simulink model "Part1_Simulink"  (R2020a)
settings: Solver=FixedStepAuto  StartTime=0.0  StopTime=inf  FixedStep=1e-3  RelTol=1e-3  EnableMultiTasking=on
undefined symbols (not defined in the file): A0, A1, D0, D1, D10, D11, D12, D13, D2, D3, D4, D5, D6, D7, D8, D9, PTA0, PTA1, PTA2, PTB2, PTB23, PTB3, PTB9, PTC16, PTC17, PTC2, PTC3, PTC4, PTD0, PTD1, PTD2, PTD3
libraries: frdmk64flib x22, nucleoutilitieslib x17
settings Model: ExtModeTrigDuration=5  Creator=kathr  LastModifiedBy=kathr
settings OptimizationCC: EnhancedBackFolding=on  PassReuseOutputArgsAs=Individual arguments  ZeroExternalMemoryAtStartup=off  ZeroInternalMemoryAtStartup=off  MaxStackSize=64  OptimizeBlockOrder=speed  DifferentSizesBufferReuse=on  OptimizationCustomize=off  EfficientTunableParamExpr=on
settings DebuggingCC: ParameterTunabilityLossMsg=error
settings HardwareCC: ProdBitPerPointer=32  ProdBitPerSizeT=32  ProdBitPerPtrDiffT=32  ProdLargestAtomicInteger=Long  ProdLargestAtomicFloat=Double  ProdWordSize=32  ProdHWDeviceType=ARM Compatible->ARM Cortex
settings SFSimCC: MATLABDynamicMemAlloc=off
settings RTWCC: SystemTargetFile=ert.tlc  HardwareBoard=NXP FRDM-K64F  TemplateMakefile=ert_default_tmf  Toolchain=GNU Tools for ARM Embedded Processors
settings CodeAppCC: ForceParamTrailComments=on  IgnoreCustomStorageClasses=off  OperatorAnnotations=on  SimulinkDataObjDesc=on  SFDataObjDesc=on  InsertBlockDesc=on

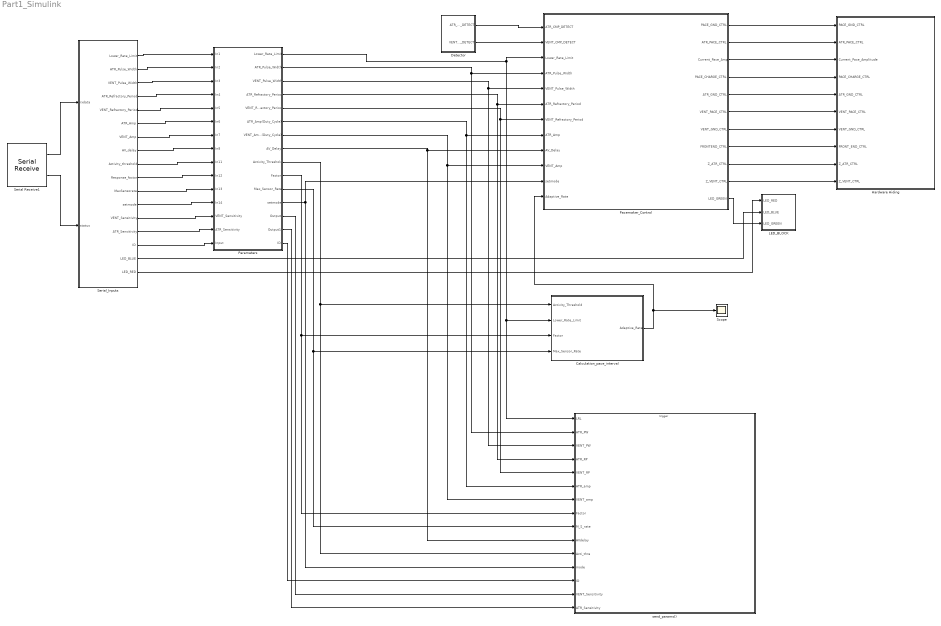
== system Part1_Simulink ==
  Calculation_pace_interval : Subsystem
  Detector : Subsystem
  Hardware Hiding : Subsystem
  LED_BLOCK : Subsystem
  Pacemaker_Control : Stateflow chart  TreatAsAtomicUnit=on
  Parameters : Subsystem
  Scope : Scope
  Serial Receive1 : frdmk64flib/Serial Receive  SCIModule=0  Baudrate=uint32(9600)  Parity=None  StopBits=1  HardwareFlowControl=None  ByteOrder=LittleEndian  DataType=uint8  DataLength=42  BlockingMode=off  OutputStatus=on  SampleTime=-1
  Serial_Inputs : Stateflow chart  TreatAsAtomicUnit=on
  "send_params() " : Subsystem
  wires:
  Serial_Inputs/7(VENT_Amp) -> Parameters/7(In7)
  Serial_Inputs/4(ATR_Refractory_Period) -> Parameters/4(In4)
  Pacemaker_Control/4(PACE_CHARGE_CTRL) -> Hardware Hiding/4(PACE_CHARGE_CTRL)
  Serial_Inputs/2(ATR_Pulse_Width) -> Parameters/2(In2)
  Parameters/4(ATR_Refractory_Period) -> "send_params() "/4(ATR_RP), Pacemaker_Control/6(ATR_Refractory_Period)
  Pacemaker_Control/9(Z_ATR_CTRL) -> Hardware Hiding/9(Z_ATR_CTRL)
  Parameters/5(VENT_Refractory_Period) -> "send_params() "/5(VENT_RP), Pacemaker_Control/7(VENT_Refractory_Period)
  Calculation_pace_interval/1(Adaptive_Rate) -> Pacemaker_Control/12(Adaptive_Rate), Scope/1
  Serial_Inputs/3(VENT_Pulse_Width) -> Parameters/3(In3)
  Pacemaker_Control/7(VENT_GND_CTRL) -> Hardware Hiding/7(VENT_GND_CTRL)
  Serial_Inputs/17(LED_RED) -> LED_BLOCK/1(LED_RED)
  Parameters/3(VENT_Pulse_Width) -> "send_params() "/3(VENT_PW), Pacemaker_Control/5(VENT_Pulse_Width)
  Detector/1(ATR_CMP_DETECT) -> Pacemaker_Control/1(ATR_CMP_DETECT)
  Pacemaker_Control/5(ATR_GND_CTRL) -> Hardware Hiding/5(ATR_GND_CTRL)
  Parameters/10(Factor) -> "send_params() "/8(Factor), Calculation_pace_interval/3(Factor)
  Parameters/8(AV_Delay) -> "send_params() "/10(AVdelay), Pacemaker_Control/9(AV_Delay)
  Pacemaker_Control/10(Z_VENT_CTRL) -> Hardware Hiding/10(Z_VENT_CTRL)
  Serial_Inputs/9(Activity_threshold) -> Parameters/9(In11)
  Parameters/1("Lower_Rate_Limit ") -> Pacemaker_Control/3(Lower_Rate_Limit), "send_params() "/1(LRL), Calculation_pace_interval/2(Lower_Rate_Limit)
  Serial_Inputs/5(VENT_Refractory_Period) -> Parameters/5(In5)
  Parameters/7(VENT_Amp(Duty_Cycle)) -> "send_params() "/7(VENT_amp), Pacemaker_Control/10(VENT_Amp)
  Serial_Inputs/11(MaxSensorate) -> Parameters/11(In13)
  Parameters/9(Activity_Threshold) -> "send_params() "/11(Acti_thre), Calculation_pace_interval/1(Activity_Threshold)
  Serial_Inputs/6(ATR_Amp) -> Parameters/6(In6)
  Pacemaker_Control/1(PACE_GND_CTRL) -> Hardware Hiding/1(PACE_GND_CTRL)
  Serial_Inputs/10(Response_factor) -> Parameters/10(In12)
  Serial_Inputs/12(setmode) -> Parameters/12(In14)
  Pacemaker_Control/3(Current_Pace_Amp) -> Hardware Hiding/3(Current_Pace_Amplitude)
  Parameters/11(Max_Sensor_Rate) -> "send_params() "/9(M_S_rate), Calculation_pace_interval/4(Max_Sensor_Rate)
  Pacemaker_Control/6(VENT_PACE_CTRL) -> Hardware Hiding/6(VENT_PACE_CTRL)
  Parameters/6(ATR_Amp(Duty_Cycle)) -> "send_params() "/6(ATR_amp), Pacemaker_Control/8(ATR_Amp)
  Pacemaker_Control/8(FRONTEND_CTRL) -> Hardware Hiding/8(FRONT_END_CTRL)
  Parameters/12("setmode ") -> "send_params() "/12(mode), Pacemaker_Control/11(setmode)
  Serial Receive1/1 -> Serial_Inputs/1(rxdata)
  Serial_Inputs/1(Lower_Rate_Limit) -> Parameters/1(In1)
  Detector/2(VENT_CMP_DETECT) -> Pacemaker_Control/2(VENT_CMP_DETECT)
  Parameters/2(ATR_Pulse_Width) -> "send_params() "/2(ATR_PW), Pacemaker_Control/4(ATR_Pulse_Width)
  Serial_Inputs/8(AV_delay) -> Parameters/8(In8)
  Pacemaker_Control/2(ATR_PACE_CTRL) -> Hardware Hiding/2(ATR_PACE_CTRL)
  Serial_Inputs/13(VENT_Sensitivity) -> Parameters/13(VENT_Sensitivity)
  Serial_Inputs/14(ATR_Sensitivity) -> Parameters/14(ATR_Sensitivity)
  Serial_Inputs/15(ID) -> Parameters/15(Input)
  Parameters/13(Output) -> "send_params() "/14(VENT_Sensitivity)
  Parameters/14(Output1) -> "send_params() "/15(ATR_Sensitivity)
  Parameters/15(ID) -> "send_params() "/13(ID)
  Serial_Inputs/16(LED_BLUE) -> LED_BLOCK/2(LED_BLUE)
  Pacemaker_Control/11(LED_GREEN) -> LED_BLOCK/3(LED_GREEN)
  Serial Receive1/2 -> Serial_Inputs/2(status)

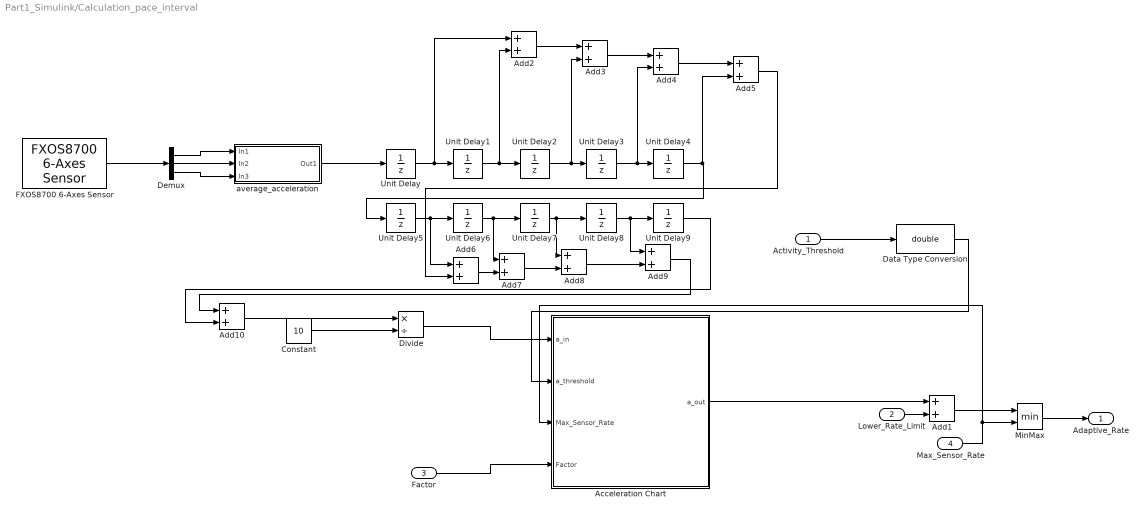
== system Part1_Simulink/Calculation_pace_interval ==
  Activity_Threshold : Inport  OutDataTypeStr=uint16
  Lower_Rate_Limit : Inport  Port=2  OutDataTypeStr=uint16
  Factor : Inport  Port=3  OutDataTypeStr=uint16
  Max_Sensor_Rate : Inport  Port=4  OutDataTypeStr=uint16
  Acceleration Chart : Stateflow chart  TreatAsAtomicUnit=on
  Add{1..10} (10 alike) : Sum
  Constant : Constant  Value=10
  Data Type Conversion : DataTypeConversion  OutDataTypeStr=double
  Demux : Demux  Outputs=3
  Divide : Product  Inputs=*/
  FXOS8700 6-Axes Sensor : frdmk64flib/FXOS8700 6-Axes Sensor  Activesensor=Accelerometer only  ODR=1.5625Hz  HybridODR=400Hz  Accelfullrange=-4g to +4g  SampleTime=0.1
  MinMax : MinMax  Inputs=2
  Unit Delay{,1..9} (10 alike) : UnitDelay  SampleTime=-1  HasFrameUpgradeWarning=on
  average_acceleration : Subsystem
  Adaptive_Rate : Outport  OutDataTypeStr=uint16  VectorParamsAs1DForOutWhenUnconnected=off
  wires:
  Lower_Rate_Limit/1 -> Add1/2
  Acceleration Chart/1(a_out) -> Add1/1
  Activity_Threshold/1 -> Data Type Conversion/1
  Factor/1 -> Acceleration Chart/4(Factor)
  Add1/1 -> MinMax/1
  MinMax/1 -> Adaptive_Rate/1
  Demux/3 -> average_acceleration/3(In3)
  Demux/1 -> average_acceleration/1(In1)
  Demux/2 -> average_acceleration/2(In2)
  FXOS8700 6-Axes Sensor/1 -> Demux/1
  Max_Sensor_Rate/1 -> MinMax/2, Acceleration Chart/3(Max_Sensor_Rate)
  Data Type Conversion/1 -> Acceleration Chart/2(a_threshold)
  Unit Delay1/1 -> Add2/2, Unit Delay2/1
  Unit Delay2/1 -> Add3/2, Unit Delay3/1
  Unit Delay3/1 -> Add4/2, Unit Delay4/1
  Unit Delay4/1 -> Add5/2, Unit Delay5/1
  Unit Delay5/1 -> Add6/1, Unit Delay6/1
  Unit Delay6/1 -> Add7/1, Unit Delay7/1
  Unit Delay7/1 -> Add8/1, Unit Delay8/1
  Unit Delay8/1 -> Add9/1, Unit Delay9/1
  Constant/1 -> Divide/2
  Divide/1 -> Acceleration Chart/1(a_in)
  average_acceleration/1(Out1) -> Unit Delay/1
  Unit Delay/1 -> Add2/1, Unit Delay1/1
  Add2/1 -> Add3/1
  Add3/1 -> Add4/1
  Add4/1 -> Add5/1
  Add5/1 -> Add6/2
  Add6/1 -> Add7/2
  Add8/1 -> Add9/2
  Add10/1 -> Divide/1
  Add9/1 -> Add10/1
  Unit Delay9/1 -> Add10/2
  Add7/1 -> Add8/2

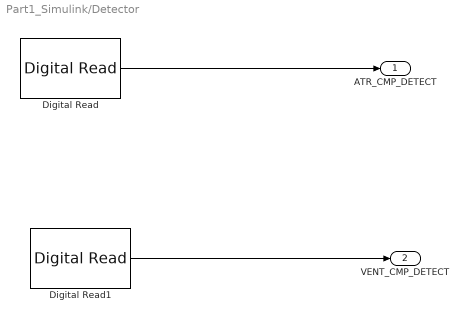
== system Part1_Simulink/Detector ==
  Digital Read : frdmk64flib/Digital Read  Whichpin=PTC16 (D0)  SampleTime=-1
  Digital Read1 : frdmk64flib/Digital Read  Whichpin=PTC17 (D1)  SampleTime=-1
  ATR_CMP_DETECT : Outport  OutDataTypeStr=boolean
  VENT_CMP_DETECT : Outport  Port=2  OutDataTypeStr=boolean
  wires:
  Digital Read/1 -> ATR_CMP_DETECT/1
  Digital Read1/1 -> VENT_CMP_DETECT/1

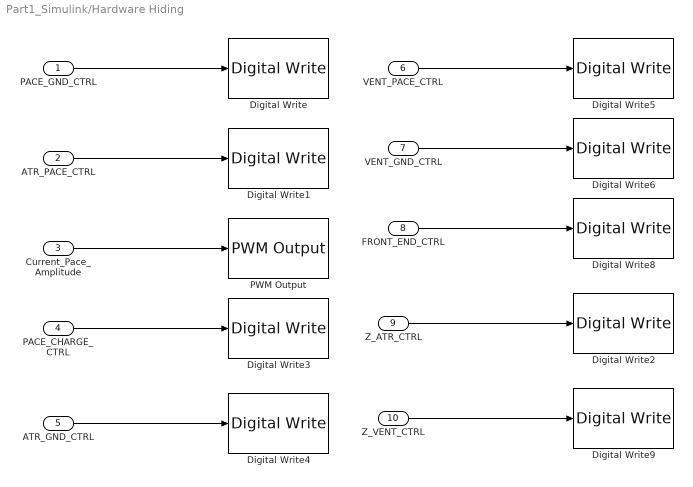
== system Part1_Simulink/Hardware Hiding ==
  PACE_GND_CTRL : Inport  OutDataTypeStr=boolean
  ATR_PACE_CTRL : Inport  Port=2  OutDataTypeStr=boolean
  Current_Pace_Amplitude : Inport  Port=3  OutDataTypeStr=uint16
  PACE_CHARGE_CTRL : Inport  Port=4  OutDataTypeStr=boolean
  ATR_GND_CTRL : Inport  Port=5  OutDataTypeStr=boolean
  VENT_PACE_CTRL : Inport  Port=6  OutDataTypeStr=boolean
  VENT_GND_CTRL : Inport  Port=7  OutDataTypeStr=boolean
  FRONT_END_CTRL : Inport  Port=8  OutDataTypeStr=boolean
  Z_ATR_CTRL : Inport  Port=9  OutDataTypeStr=boolean
  Z_VENT_CTRL : Inport  Port=10  OutDataTypeStr=boolean
  Digital Write : frdmk64flib/Digital Write  Whichpin=PTD0 (D10)
  Digital Write1 : frdmk64flib/Digital Write  Whichpin=PTA0 (D8)
  Digital Write2 : frdmk64flib/Digital Write  Whichpin=PTB23 (D4)
  Digital Write3 : frdmk64flib/Digital Write  Whichpin=PTB9 (D2)
  Digital Write4 : frdmk64flib/Digital Write  Whichpin=PTD2 (D11)
  Digital Write5 : frdmk64flib/Digital Write  Whichpin=PTC4 (D9)
  Digital Write6 : frdmk64flib/Digital Write  Whichpin=PTD3 (D12)
  Digital Write8 : frdmk64flib/Digital Write  Whichpin=PTD1 (D13)
  Digital Write9 : frdmk64flib/Digital Write  Whichpin=PTC3 (D7)
  PWM Output : frdmk64flib/PWM Output  Whichpin=PTA2 (D5)  InitialFrequency=2000  InitialDutyCycle=100
  wires:
  PACE_GND_CTRL/1 -> Digital Write/1
  ATR_PACE_CTRL/1 -> Digital Write1/1
  Current_Pace_Amplitude/1 -> PWM Output/1
  PACE_CHARGE_CTRL/1 -> Digital Write3/1
  ATR_GND_CTRL/1 -> Digital Write4/1
  VENT_PACE_CTRL/1 -> Digital Write5/1
  VENT_GND_CTRL/1 -> Digital Write6/1
  FRONT_END_CTRL/1 -> Digital Write8/1
  Z_VENT_CTRL/1 -> Digital Write9/1
  Z_ATR_CTRL/1 -> Digital Write2/1

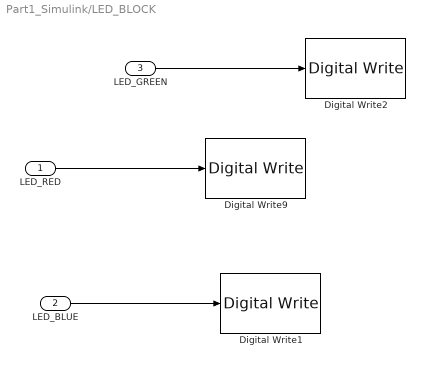
== system Part1_Simulink/LED_BLOCK ==
  LED_RED : Inport  OutDataTypeStr=boolean
  LED_BLUE : Inport  Port=2  OutDataTypeStr=boolean
  LED_GREEN : Inport  Port=3  OutDataTypeStr=boolean
  Digital Write1 : frdmk64flib/Digital Write  Whichpin=BLUE_LED
  Digital Write2 : frdmk64flib/Digital Write  Whichpin=GREEN_LED
  Digital Write9 : frdmk64flib/Digital Write  Whichpin=RED_LED
  wires:
  LED_RED/1 -> Digital Write9/1
  LED_BLUE/1 -> Digital Write1/1
  LED_GREEN/1 -> Digital Write2/1

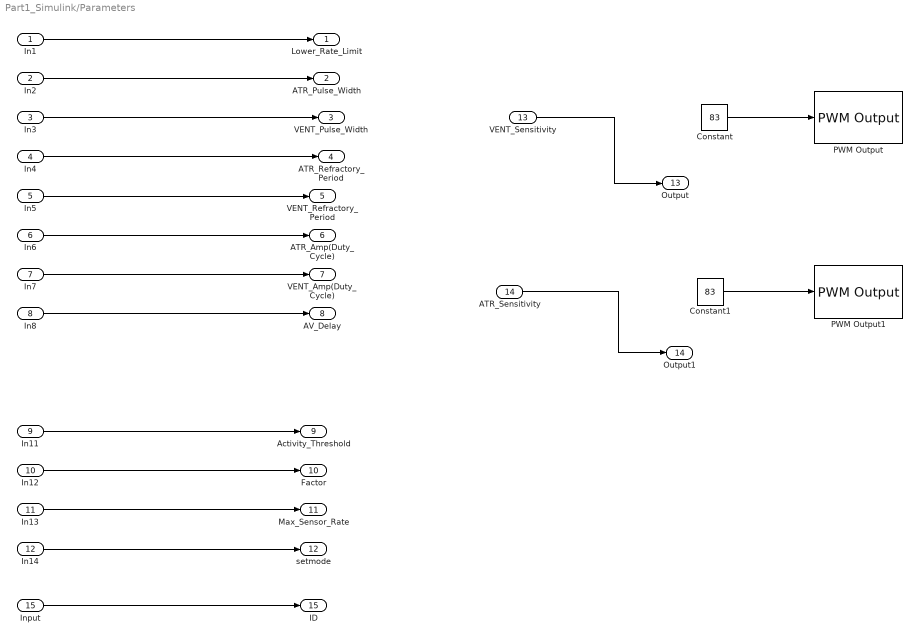
== system Part1_Simulink/Parameters ==
  In1 : Inport
  In2 : Inport  Port=2
  In3 : Inport  Port=3
  In4 : Inport  Port=4
  In5 : Inport  Port=5
  In6 : Inport  Port=6
  In7 : Inport  Port=7
  In8 : Inport  Port=8
  In11 : Inport  Port=9
  In12 : Inport  Port=10
  In13 : Inport  Port=11
  In14 : Inport  Port=12
  VENT_Sensitivity : Inport  Port=13
  ATR_Sensitivity : Inport  Port=14
  Input : Inport  Port=15
  Constant : Constant  Value=83
  Constant1 : Constant  Value=83
  PWM Output : frdmk64flib/PWM Output  Whichpin=PTC2 (D6)  InitialFrequency=2000  InitialDutyCycle=75
  PWM Output1 : frdmk64flib/PWM Output  Whichpin=PTA1 (D3)  InitialFrequency=2000  InitialDutyCycle=100
  "Lower_Rate_Limit " : Outport  OutDataTypeStr=uint16
  ATR_Pulse_Width : Outport  Port=2  OutDataTypeStr=uint16
  VENT_Pulse_Width : Outport  Port=3  OutDataTypeStr=uint16
  ATR_Refractory_Period : Outport  Port=4  OutDataTypeStr=uint16
  VENT_Refractory_Period : Outport  Port=5  OutDataTypeStr=uint16
  ATR_Amp(Duty_Cycle) : Outport  Port=6  OutDataTypeStr=uint16
  VENT_Amp(Duty_Cycle) : Outport  Port=7  OutDataTypeStr=uint16
  AV_Delay : Outport  Port=8  OutDataTypeStr=uint16
  Activity_Threshold : Outport  Port=9  OutDataTypeStr=uint16
  Factor : Outport  Port=10  OutDataTypeStr=uint16
  Max_Sensor_Rate : Outport  Port=11  OutDataTypeStr=uint16
  "setmode " : Outport  Port=12  VectorParamsAs1DForOutWhenUnconnected=off
  Output : Outport  Port=13
  Output1 : Outport  Port=14
  ID : Outport  Port=15
  wires:
  In5/1 -> VENT_Refractory_Period/1
  In2/1 -> ATR_Pulse_Width/1
  In4/1 -> ATR_Refractory_Period/1
  In6/1 -> ATR_Amp(Duty_Cycle)/1
  In7/1 -> VENT_Amp(Duty_Cycle)/1
  In3/1 -> VENT_Pulse_Width/1
  In1/1 -> "Lower_Rate_Limit "/1
  In8/1 -> AV_Delay/1
  In11/1 -> Activity_Threshold/1
  In12/1 -> Factor/1
  In13/1 -> Max_Sensor_Rate/1
  In14/1 -> "setmode "/1
  Input/1 -> ID/1
  VENT_Sensitivity/1 -> Output/1
  ATR_Sensitivity/1 -> Output1/1
  Constant/1 -> PWM Output/1
  Constant1/1 -> PWM Output1/1

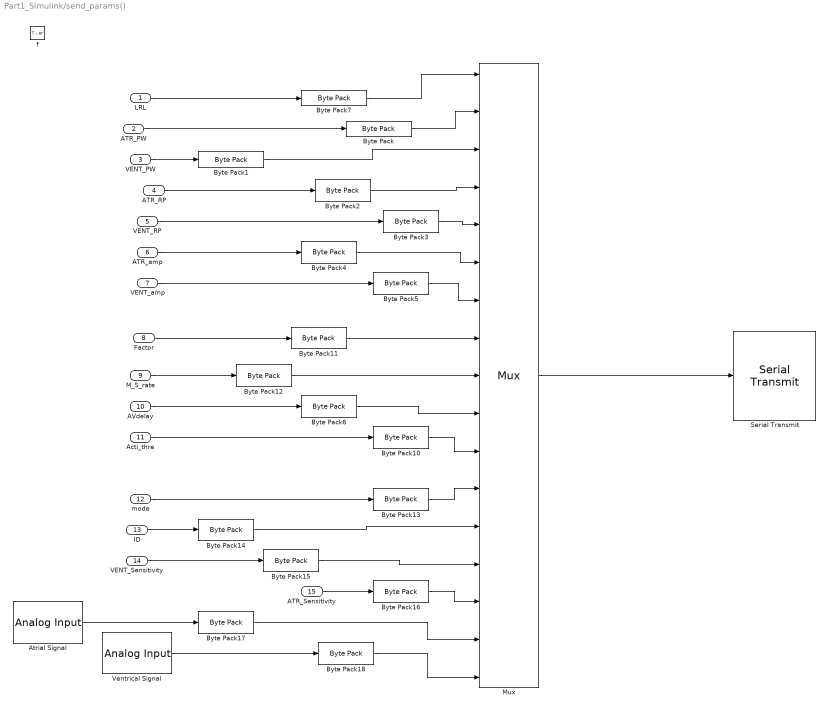
== system Part1_Simulink/send_params()  ==
  LRL : Inport  OutDataTypeStr=uint16
  ATR_PW : Inport  Port=2  OutDataTypeStr=uint16
  VENT_PW : Inport  Port=3  OutDataTypeStr=uint16
  ATR_RP : Inport  Port=4  OutDataTypeStr=uint16
  VENT_RP : Inport  Port=5  OutDataTypeStr=uint16
  ATR_amp : Inport  Port=6  OutDataTypeStr=uint16
  VENT_amp : Inport  Port=7  OutDataTypeStr=uint16
  Factor : Inport  Port=8  OutDataTypeStr=uint16
  M_S_rate : Inport  Port=9  OutDataTypeStr=uint16
  AVdelay : Inport  Port=10  OutDataTypeStr=uint16
  Acti_thre : Inport  Port=11  OutDataTypeStr=uint16
  mode : Inport  Port=12  OutDataTypeStr=uint16
  ID : Inport  Port=13  OutDataTypeStr=uint16
  VENT_Sensitivity : Inport  Port=14  OutDataTypeStr=double
  ATR_Sensitivity : Inport  Port=15  OutDataTypeStr=double
  f : TriggerPort  TriggerType=function-call  IsSimulinkFunction=on  FunctionName=send_params  VariantControl=(inherit)
  Atrial Signal : frdmk64flib/Analog Input  Whichpin=PTB2 (A0)  SampleTime=-1
  Byte Pack{,1..7,10..14} (13 alike) : nucleoutilitieslib/Byte Pack  datatypes={'uint16'}  byteAlign=1  blockPlatform=nucleo
      settings: SourceProductBaseCode=ARDUINO,ML_ARDUINO,ECCORTEXA,ECCORTEXR,SC_BEAGLEBONE_BLUE,EC_FREEDOM_BOARD,EC_FRDM_K64F,INTEL_BLOCKSET,MICROBIT,NUCLEO,PX4AUTOPILOTS,RASPPIIO,STMICRODIS,TIC2000,XILINX_BLOCKSET
  Byte Pack{15..18} (4 alike) : nucleoutilitieslib/Byte Pack  datatypes={'double'}  byteAlign=1  blockPlatform=nucleo
      settings: SourceProductBaseCode=ARDUINO,ML_ARDUINO,ECCORTEXA,ECCORTEXR,SC_BEAGLEBONE_BLUE,EC_FREEDOM_BOARD,EC_FRDM_K64F,INTEL_BLOCKSET,MICROBIT,NUCLEO,PX4AUTOPILOTS,RASPPIIO,STMICRODIS,TIC2000,XILINX_BLOCKSET
  Mux : Mux  Inputs=17
  Serial Transmit : frdmk64flib/Serial Transmit  SCIModule=0  Baudrate=uint32(9600)  Parity=None  StopBits=1  HardwareFlowControl=None  ByteOrder=LittleEndian  BlockingMode=on  OutputStatus=off
  Ventrical Signal : frdmk64flib/Analog Input  Whichpin=PTB3 (A1)  SampleTime=-1
  wires:
  LRL/1 -> Byte Pack7/1
  VENT_PW/1 -> Byte Pack1/1
  ATR_RP/1 -> Byte Pack2/1
  Mux/1 -> Serial Transmit/1
  ATR_amp/1 -> Byte Pack4/1
  VENT_RP/1 -> Byte Pack3/1
  VENT_amp/1 -> Byte Pack5/1
  ATR_PW/1 -> Byte Pack/1
  Byte Pack/1 -> Mux/2
  Byte Pack1/1 -> Mux/3
  Byte Pack2/1 -> Mux/4
  Byte Pack3/1 -> Mux/5
  Byte Pack4/1 -> Mux/6
  Byte Pack5/1 -> Mux/7
  Byte Pack7/1 -> Mux/1
  AVdelay/1 -> Byte Pack6/1
  Acti_thre/1 -> Byte Pack10/1
  Factor/1 -> Byte Pack11/1
  M_S_rate/1 -> Byte Pack12/1
  mode/1 -> Byte Pack13/1
  ID/1 -> Byte Pack14/1
  VENT_Sensitivity/1 -> Byte Pack15/1
  ATR_Sensitivity/1 -> Byte Pack16/1
  Atrial Signal/1 -> Byte Pack17/1
  Ventrical Signal/1 -> Byte Pack18/1
  Byte Pack11/1 -> Mux/8
  Byte Pack12/1 -> Mux/9
  Byte Pack6/1 -> Mux/10
  Byte Pack10/1 -> Mux/11
  Byte Pack13/1 -> Mux/12
  Byte Pack14/1 -> Mux/13
  Byte Pack15/1 -> Mux/14
  Byte Pack16/1 -> Mux/15
  Byte Pack17/1 -> Mux/16
  Byte Pack18/1 -> Mux/17

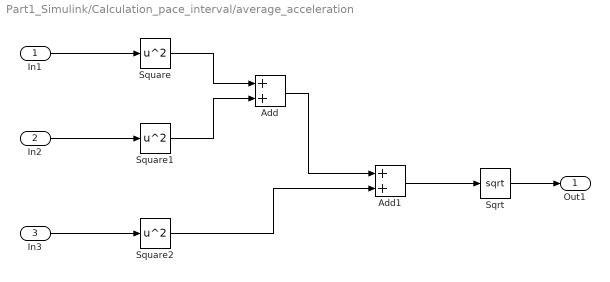
== system Part1_Simulink/Calculation_pace_interval/average_acceleration ==
  In1 : Inport
  In2 : Inport  Port=2
  In3 : Inport  Port=3
  Add : Sum
  Add1 : Sum
  Sqrt : Sqrt  SaturateOnIntegerOverflow=on
  Square : Math  Operator=square  SignedPower=on  SaturateOnIntegerOverflow=on
  Square1 : Math  Operator=square  SignedPower=on  SaturateOnIntegerOverflow=on
  Square2 : Math  Operator=square  SignedPower=on  SaturateOnIntegerOverflow=on
  Out1 : Outport
  wires:
  In1/1 -> Square/1
  In2/1 -> Square1/1
  In3/1 -> Square2/1
  Square/1 -> Add/1
  Square1/1 -> Add/2
  Add/1 -> Add1/1
  Square2/1 -> Add1/2
  Add1/1 -> Sqrt/1
  Sqrt/1 -> Out1/1

== stateflow chart Part1_Simulink/Calculation_pace_interval/Acceleration Chart ==
  state LOW_TO_MID
    entry:
    if(a_out+Factor<=Max_Sensor_Rate/2)
    a_out = a_out + Factor;
    end
  state MID
    entry:
    %LED_BLUE = true;
  state LOW
    entry:
    a_out = 0;
    %LED_RED = true;
  state MID_TO_HIGH
    entry:
    if(a_out+Factor <=Max_Sensor_Rate)
    a_out = a_out+Factor;
    end
  state LOW_TO_HIGH
    entry:
    if(a_out+Factor+Factor <=Max_Sensor_Rate)
    a_out = a_out+Factor+Factor;
    end
  state HIGH_TO_MID
    entry:
    a_out = a_out-Factor;
  state HIGH
    entry:
    %LED_BLUE = true;
  LOW_TO_MID -> MID
  LOW -> LOW_TO_MID [order 2] : [a_in<=(1+a_threshold/10) && a_in>(1+a_threshold/20)]
  MID -> MID [order 1] : [a_in<=(1+a_threshold/10) && a_in>(1+a_threshold/20)]
  HIGH_TO_MID -> MID
  (default) -> LOW
  MID -> LOW [order 2] : [a_in<=(1+a_threshold/20)]
  MID -> MID_TO_HIGH [order 3] : [a_in>(1+a_threshold/10)]
  LOW -> LOW [order 1] : [a_in<=(1+a_threshold/20)]
  LOW -> LOW_TO_HIGH [order 3] : [a_in>(1+a_threshold/10)]
  HIGH -> LOW [order 2] : [a_in<=(1+a_threshold/20)]
  MID_TO_HIGH -> HIGH
  HIGH -> HIGH [order 1] : [a_in>(1+a_threshold/10)]
  LOW_TO_HIGH -> HIGH
  HIGH -> HIGH_TO_MID [order 3] : [a_in<=(1+a_threshold/5) && a_in>(1+a_threshold/20)]
  data: a_in input double; a_out output uint16; a_threshold input double; Max_Sensor_Rate input uint16; Factor input uint16

== stateflow chart Part1_Simulink/Pacemaker_Control ==
  state AOO
    entry:
    PACE_CHARGE_CTRL=false;
    VENT_PACE_CTRL=false;
    PACE_CHARGE_CTRL=true;
    PACE_GND_CTRL=true;
    VENT_PACE_CTRL=false;
    Z_ATR_CTRL=false;
    Z_VENT_CTRL=false;
    ATR_PACE_CTRL=false;
    ATR_GND_CTRL=true;
    VENT_GND_CTRL=false;
    %LED_GREEN=false;
  state AOO_PACE
    entry:
    PACE_CHARGE_CTRL=false;
    PACE_GND_CTRL=true;
    ATR_PACE_CTRL=true;
    ATR_GND_CTRL=false;
    Z_ATR_CTRL=false;
    Z_VENT_CTRL=false;
    VENT_GND_CTRL=false;
    VENT_PACE_CTRL=false;
    %LED_GREEN=true;
    Current_Pace_Amp=ATR_Amp;
  state AOOR
    entry:
    PACE_CHARGE_CTRL=false;
    VENT_PACE_CTRL=false;
    PACE_CHARGE_CTRL=true;
    PACE_GND_CTRL=true;
    VENT_PACE_CTRL=false;
    Z_ATR_CTRL=false;
    Z_VENT_CTRL=false;
    ATR_PACE_CTRL=false;
    ATR_GND_CTRL=true;
    VENT_GND_CTRL=false;
    LED_GREEN=false;
  state pacing_AOOR
    entry:
    PACE_CHARGE_CTRL=false;
    PACE_GND_CTRL=true;
    ATR_PACE_CTRL=true;
    ATR_GND_CTRL=false;
    Z_ATR_CTRL=false;
    Z_VENT_CTRL=false;
    VENT_GND_CTRL=false;
    VENT_PACE_CTRL=false;
    LED_GREEN=true;
    Current_Pace_Amp=ATR_Amp;
  state VOO_PACE
    entry:
    PACE_CHARGE_CTRL=false;
    PACE_GND_CTRL=true;
    ATR_PACE_CTRL=false;
    ATR_GND_CTRL=false;
    Z_ATR_CTRL=false;
    Z_VENT_CTRL=false;
    VENT_GND_CTRL=false;
    VENT_PACE_CTRL=true;
    %LED_GREEN=true;
    Current_Pace_Amp = VENT_Amp;
  state VOO
    entry:
    PACE_CHARGE_CTRL=false;
    VENT_PACE_CTRL=false;
    PACE_CHARGE_CTRL=true;
    PACE_GND_CTRL=true;
    VENT_PACE_CTRL=false;
    Z_ATR_CTRL=false;
    Z_VENT_CTRL=false;
    ATR_PACE_CTRL=false;
    ATR_GND_CTRL=false;
    VENT_GND_CTRL=true;
    %LED_GREEN=false;
  state VOOR
    entry:
    PACE_CHARGE_CTRL=false;
    VENT_PACE_CTRL=false;
    PACE_CHARGE_CTRL=true;
    PACE_GND_CTRL=true;
    VENT_PACE_CTRL=false;
    Z_ATR_CTRL=false;
    Z_VENT_CTRL=false;
    ATR_PACE_CTRL=false;
    ATR_GND_CTRL=false;
    VENT_GND_CTRL=true;
    LED_GREEN=false;
  state pacing_VOOR
    entry:
    PACE_CHARGE_CTRL=false;
    PACE_GND_CTRL=true;
    ATR_PACE_CTRL=false;
    ATR_GND_CTRL=false;
    Z_ATR_CTRL=false;
    Z_VENT_CTRL=false;
    VENT_GND_CTRL=false;
    VENT_PACE_CTRL=true;
    LED_GREEN=true;
    Current_Pace_Amp = VENT_Amp;
  state AAI_PACE
    entry:
    FRONTEND_CTRL=false;
    PACE_CHARGE_CTRL=false;
    PACE_GND_CTRL=true;
    ATR_PACE_CTRL=true;
    ATR_GND_CTRL=false;
    Z_ATR_CTRL=false;
    Z_VENT_CTRL=false;
    VENT_GND_CTRL=false;
    VENT_PACE_CTRL=false;
    %LED_GREEN=true;
    Current_Pace_Amp=ATR_Amp;
  state AAI
    entry:
    FRONTEND_CTRL=false;
    PACE_CHARGE_CTRL=false;
    VENT_PACE_CTRL=false;
    PACE_CHARGE_CTRL=true;
    PACE_GND_CTRL=true;
    VENT_PACE_CTRL=false;
    Z_ATR_CTRL=false;
    Z_VENT_CTRL=false;
    ATR_PACE_CTRL=false;
    ATR_GND_CTRL=true;
    VENT_GND_CTRL=false;
    %LED_GREEN=false;
  state AAI_REF_PERIOD1
    entry:
    FRONTEND_CTRL=true;
    PACE_CHARGE_CTRL=true;
    PACE_GND_CTRL=true;
    ATR_PACE_CTRL=false;
    ATR_GND_CTRL=true;
    Z_ATR_CTRL=false;
    Z_VENT_CTRL=false;
    VENT_GND_CTRL=false;
    VENT_PACE_CTRL=false;
    %LED_GREEN=true;
    Current_Pace_Amp=ATR_Amp;
  state pacing_AAIR
    entry:
    FRONTEND_CTRL=false;
    PACE_CHARGE_CTRL=false;
    PACE_GND_CTRL=true;
    ATR_PACE_CTRL=true;
    ATR_GND_CTRL=false;
    Z_ATR_CTRL=false;
    Z_VENT_CTRL=false;
    VENT_GND_CTRL=false;
    VENT_PACE_CTRL=false;
    %LED_GREEN=true;
    Current_Pace_Amp=ATR_Amp;
  state AAIR
    entry:
    FRONTEND_CTRL=false;
    PACE_CHARGE_CTRL=false;
    VENT_PACE_CTRL=false;
    PACE_CHARGE_CTRL=true;
    PACE_GND_CTRL=true;
    VENT_PACE_CTRL=false;
    Z_ATR_CTRL=false;
    Z_VENT_CTRL=false;
    ATR_PACE_CTRL=false;
    ATR_GND_CTRL=true;
    VENT_GND_CTRL=false;
    %LED_GREEN=false;
  state AAI_REF_LED1
    entry:
    %LED_GREEN=false;
  state AAIR_LED1
    entry:
    %LED_GREEN=false;
  state AAI_REF_PERIOD
    entry:
    FRONTEND_CTRL=true;
    PACE_CHARGE_CTRL=true;
    PACE_GND_CTRL=true;
    ATR_PACE_CTRL=false;
    ATR_GND_CTRL=true;
    Z_ATR_CTRL=false;
    Z_VENT_CTRL=false;
    VENT_GND_CTRL=false;
    VENT_PACE_CTRL=false;
    %LED_GREEN=true;
    Current_Pace_Amp=ATR_Amp;
  state Refractory_AAIR1
    entry:
    FRONTEND_CTRL=true;
    PACE_CHARGE_CTRL=true;
    PACE_GND_CTRL=true;
    ATR_PACE_CTRL=false;
    ATR_GND_CTRL=true;
    Z_ATR_CTRL=false;
    Z_VENT_CTRL=false;
    VENT_GND_CTRL=false;
    VENT_PACE_CTRL=false;
    %LED_GREEN=true;
    Current_Pace_Amp=ATR_Amp
  state AAI_REF_LED
    entry:
    %LED_GREEN=false;
  state MAIN
    entry:
    %stop sensing
    FRONTEND_CTRL=false;
    Current_Pace_Amp=0;
  state VVI
    entry:
    FRONTEND_CTRL=false;
    PACE_CHARGE_CTRL=false;
    VENT_PACE_CTRL=false;
    PACE_CHARGE_CTRL=true;
    PACE_GND_CTRL=true;
    VENT_PACE_CTRL=false;
    Z_ATR_CTRL=false;
    Z_VENT_CTRL=false;
    ATR_PACE_CTRL=false;
    ATR_GND_CTRL=false;
    VENT_GND_CTRL=true;
    LED_GREEN=false;
  state Refractory_AAIR
    entry:
    FRONTEND_CTRL=true;
    PACE_CHARGE_CTRL=true;
    PACE_GND_CTRL=true;
    ATR_PACE_CTRL=false;
    ATR_GND_CTRL=true;
    Z_ATR_CTRL=false;
    Z_VENT_CTRL=false;
    VENT_GND_CTRL=false;
    VENT_PACE_CTRL=false;
    %LED_GREEN=true;
    Current_Pace_Amp=ATR_Amp
  state VVI_PACE
    entry:
    FRONTEND_CTRL=false;
    PACE_CHARGE_CTRL=false;
    PACE_GND_CTRL=true;
    ATR_PACE_CTRL=false;
    ATR_GND_CTRL=false;
    Z_ATR_CTRL=false;
    Z_VENT_CTRL=false;
    VENT_GND_CTRL=false;
    VENT_PACE_CTRL=true;
    LED_GREEN=true;
    Current_Pace_Amp = VENT_Amp;
  note: MODE
      | NUMBER
      |
      | VOO
      | 0
      |
      | AOO
      | 1
      |
      | VVI
      | 2
      |
      | AAI
      | 3
      |
      | DOO
      | 4
      |
      | VOOR
      | 5
      |
      | AOOR
      | 6
      |
      | VVIR
      | 7
      |
      | AAIR
      | 8
      |
      | DOOR
      | 9
  state AAIR_LED
    entry:
    %LED_GREEN=false;
  state VVIR
    entry:
    FRONTEND_CTRL=false;
    PACE_CHARGE_CTRL=false;
    VENT_PACE_CTRL=false;
    PACE_CHARGE_CTRL=true;
    PACE_GND_CTRL=true;
    VENT_PACE_CTRL=false;
    Z_ATR_CTRL=false;
    Z_VENT_CTRL=false;
    ATR_PACE_CTRL=false;
    ATR_GND_CTRL=false;
    VENT_GND_CTRL=true;
    %LED_GREEN=false;
  state pacing_VVIR
    entry:
    FRONTEND_CTRL=false;
    PACE_CHARGE_CTRL=false;
    PACE_GND_CTRL=true;
    ATR_PACE_CTRL=false;
    ATR_GND_CTRL=false;
    Z_ATR_CTRL=false;
    Z_VENT_CTRL=false;
    VENT_GND_CTRL=false;
    VENT_PACE_CTRL=true;
    %LED_GREEN=true;
    Current_Pace_Amp = VENT_Amp;
  state VVI_REF_PERIOD2
    entry:
    FRONTEND_CTRL=true;
    PACE_CHARGE_CTRL=true;
    PACE_GND_CTRL=true;
    ATR_PACE_CTRL=false;
    ATR_GND_CTRL=false;
    Z_ATR_CTRL=false;
    Z_VENT_CTRL=false;
    VENT_GND_CTRL=true;
    VENT_PACE_CTRL=false;
    Current_Pace_Amp = VENT_Amp;
    LED_GREEN=false;
  state VVIR_REF_PERIOD2
    %LED_GREEN=false;
  state VVI_LED1
    entry:
    LED_GREEN=true;
  state VVI_REF_PERIOD1
    entry:
    FRONTEND_CTRL=true;
    PACE_CHARGE_CTRL=true;
    PACE_GND_CTRL=true;
    ATR_PACE_CTRL=false;
    ATR_GND_CTRL=false;
    Z_ATR_CTRL=false;
    Z_VENT_CTRL=false;
    VENT_GND_CTRL=true;
    VENT_PACE_CTRL=false;
    Current_Pace_Amp = VENT_Amp;
    LED_GREEN=false;
  state Refractory_VVIR1
    entry:
    FRONTEND_CTRL=true;
    PACE_CHARGE_CTRL=true;
    PACE_GND_CTRL=true;
    ATR_PACE_CTRL=false;
    ATR_GND_CTRL=false;
    Z_ATR_CTRL=false;
    Z_VENT_CTRL=false;
    VENT_GND_CTRL=true;
    VENT_PACE_CTRL=false;
    %LED_GREEN=true;
    Current_Pace_Amp = VENT_Amp;
  state Refractory_VVIR
    entry:
    FRONTEND_CTRL=true;
    PACE_CHARGE_CTRL=true;
    PACE_GND_CTRL=true;
    ATR_PACE_CTRL=false;
    ATR_GND_CTRL=false;
    Z_ATR_CTRL=false;
    Z_VENT_CTRL=false;
    VENT_GND_CTRL=true;
    VENT_PACE_CTRL=false;
    %LED_GREEN=true;
    Current_Pace_Amp = VENT_Amp;
  state VVI_LED
    entry:
    LED_GREEN=true;
  note: Discharge C22 to C21 to pace ATR
  state pacing_DOO_ATR
    entry:
    %discharge C22 and charge C21
    PACE_CHARGE_CTRL=false;%disconnect 4
    %connect C22 and C21
    ATR_GND_CTRL = false;
    VENT_GND_CTRL=false;%disconnect 7
    VENT_PACE_CTRL=false;
    ATR_PACE_CTRL=true;%connect 6 for ATR
    PACE_GND_CTRL=true;
    Current_Pace_Amp = ATR_Amp;
    %LED_RED=false;
  state VVIR_REF_PERIOD1
    %LED_GREEN=false;
  note: Charge C22, discharge C21 for VENT
  state DOO
    entry:
    FRONTEND_CTRL=false;
    VENT_PACE_CTRL=false %turn off VENT
    ATR_PACE_CTRL=false;%disconnect 6
    %discharge C21 for VENT
    VENT_GND_CTRL=true;
    PACE_GND_CTRL=true;%connect 10
    ATR_GND_CTRL=false;
    %charge C22
    PACE_CHARGE_CTRL=true;%connect 4
    %set the atrium pacing amplitude
    Current_Pace_Amp = ATR_Amp;
    %LED_RED=true;%use red LED for debugging
    %LED_GREEN=false;
  state pacing_DOOR_ATR
    entry:
    %discharge C22 and charge C21
    PACE_CHARGE_CTRL=false;%disconnect 4
    %connect C22 and C21
    ATR_GND_CTRL = false;
    VENT_GND_CTRL=false;%disconnect 7
    VENT_PACE_CTRL=false;
    ATR_PACE_CTRL=true;%connect 6 for ATR
    PACE_GND_CTRL=true;
    Current_Pace_Amp = ATR_Amp;
    %LED_RED=false;
  state DOOR
    entry:
    FRONTEND_CTRL=false;
    VENT_PACE_CTRL=false; %turn off VENT
    ATR_PACE_CTRL=false;%disconnect 6
    %discharge C21 for VENT
    VENT_GND_CTRL=true;
    PACE_GND_CTRL=true;%connect 10
    ATR_GND_CTRL=false;
    %charge C22
    PACE_CHARGE_CTRL=true;%connect 4
    %set the atrium pacing amplitude
    Current_Pace_Amp = ATR_Amp;
    %LED_RED=true;%use red LED for debugging
  state DOO_VENT
    entry:
    PACE_CHARGE_CTRL=false;%disconnect 4
    PACE_GND_CTRL=true;%connect 10
    VENT_GND_CTRL=false;
    VENT_PACE_CTRL=true;%connect 6
    ATR_GND_CTRL=false;%disconnect 7
    %set the ventricle pacing amplitude
    Current_Pace_Amp = VENT_Amp;
    %LED_GREEN=false;%use red LED for debugging
  state DOO_Vcharge_Adischarge
    entry:
    PACE_CHARGE_CTRL=true;%connect 4
    %disconnect C21 with C22
    ATR_PACE_CTRL=false;%disconnect 6
    VENT_PACE_CTRL=false;
    %discharge C21
    ATR_GND_CTRL=true;%connect 7
    PACE_GND_CTRL=true;%connect 10
    VENT_GND_CTRL=false;
    %set the atrium pacing amplitude
    Current_Pace_Amp = VENT_Amp;
    %LED_GREEN=false;%use green LED for debugging
  note: Discharge C22 to C21 to pace VENT
  note: Charge C22, discharge C21 for ATR
  state DOOR_Vcharge_Adischarge
    entry:
    PACE_CHARGE_CTRL=true;%connect 4
    %disconnect C21 with C22
    ATR_PACE_CTRL=false;%disconnect 6
    VENT_PACE_CTRL=false;
    %discharge C21
    ATR_GND_CTRL=true;%connect 7
    PACE_GND_CTRL=true;%connect 10
    VENT_GND_CTRL=false;
    %set the atrium pacing amplitude
    Current_Pace_Amp = VENT_Amp;
    %LED_GREEN=true;%use green LED for debugging
  state DOOR_VENT
    entry:
    PACE_CHARGE_CTRL=false;%disconnect 4
    PACE_GND_CTRL=true;%connect 10
    VENT_GND_CTRL=false;
    VENT_PACE_CTRL=true;%connect 6
    ATR_GND_CTRL=false;%disconnect 7
    %set the ventricle pacing amplitude
    Current_Pace_Amp = VENT_Amp;
    %LED_GREEN=false;%use red LED for debugging
  AOO_PACE -> AOO : after(ATR_Pulse_Width,msec)
  AOO -> MAIN [order 2] : [setmode~=1]
  AOOR -> pacing_AOOR [order 1] : after(60000/Adaptive_Rate - ATR_Pulse_Width,msec)
  AOO -> AOO_PACE [order 1] : after(60000/Lower_Rate_Limit - ATR_Pulse_Width,msec)
  MAIN -> AOO [order 2] : [setmode==1]
  pacing_AOOR -> AOOR : after(ATR_Pulse_Width,msec)
  AOOR -> MAIN [order 2] : [setmode~=6]
  MAIN -> AOOR [order 9] : [setmode==6]
  VOO -> VOO_PACE [order 1] : after(60000/Lower_Rate_Limit - VENT_Pulse_Width,msec)
  VOO_PACE -> VOO : after(VENT_Pulse_Width,msec)
  VOO -> MAIN [order 2] : [setmode~=0]
  VOOR -> pacing_VOOR [order 1] : after(60000/Adaptive_Rate - VENT_Pulse_Width,msec)
  MAIN -> VOO [order 5] : [setmode==0]
  pacing_VOOR -> VOOR : after(VENT_Pulse_Width,msec)
  AAI -> AAI_PACE [order 2]
  MAIN -> VOOR [order 3] : [setmode==5]
  VOOR -> MAIN [order 2] : [setmode~=5]
  AAI -> MAIN [order 1] : [setmode~=3]
  MAIN -> AAI [order 7] : [setmode==3]
  AAI_PACE -> AAI_REF_PERIOD : after(ATR_Pulse_Width,msec)
  AAIR -> pacing_AAIR [order 2]
  AAI_REF_PERIOD1 -> AAI_REF_LED1 : after(ATR_Refractory_Period,msec)
  MAIN -> AAIR [order 6] : [setmode==8]
  AAI_REF_LED1 -> AAI [order 2] : after(60000/Lower_Rate_Limit-ATR_Refractory_Period,msec)
  AAI_REF_LED1 -> AAI_REF_PERIOD1 [order 1] : [ATR_CMP_DETECT==true]
  AAI_REF_LED -> AAI [order 1] : after(60000/Lower_Rate_Limit-ATR_Refractory_Period-ATR_Pulse_Width,msec)
  AAIR_LED1 -> Refractory_AAIR1 [order 1] : [ATR_CMP_DETECT==true]
  AAIR -> MAIN [order 1] : [setmode~=8]
  Refractory_AAIR1 -> AAIR_LED1 : after(ATR_Refractory_Period,msec)
  AAIR_LED1 -> AAIR [order 2] : after(60000/Adaptive_Rate-ATR_Refractory_Period,msec)
  AAI_REF_LED -> AAI_REF_PERIOD1 [order 2] : [ATR_CMP_DETECT==true]
  pacing_AAIR -> Refractory_AAIR : after(ATR_Pulse_Width,msec)
  AAIR_LED -> AAIR [order 1] : after(60000/Adaptive_Rate-ATR_Refractory_Period-ATR_Pulse_Width,msec)
  (default) -> MAIN
  AAI_REF_PERIOD -> AAI_REF_LED : after(ATR_Refractory_Period,msec)
  VVIR -> MAIN [order 1] : [setmode~=7]
  VVI -> VVI_PACE [order 2]
  VVI -> MAIN [order 1] : [setmode~=2]
  MAIN -> VVIR [order 4] : [setmode==7]
  MAIN -> VVI [order 8] : [setmode==2]
  AAIR_LED -> Refractory_AAIR1 [order 2] : [ATR_CMP_DETECT==true]
  DOOR -> MAIN [order 2] : [setmode~=9]
  MAIN -> DOOR [order 10] : [setmode==9]
  DOO -> MAIN [order 2] : [setmode~=4]
  MAIN -> DOO [order 1] : [setmode==4]
  Refractory_AAIR -> AAIR_LED : after(ATR_Refractory_Period,msec)
  VVI_PACE -> VVI_REF_PERIOD1 : after(VENT_Pulse_Width,msec)
  VVI_LED -> VVI [order 2] : after(60000/Lower_Rate_Limit-VENT_Refractory_Period-VENT_Pulse_Width,msec)
  VVI_LED1 -> VVI [order 1] : after(60000/Lower_Rate_Limit-VENT_Refractory_Period,msec)
  VVIR -> pacing_VVIR [order 2]
  VVI_LED1 -> VVI_REF_PERIOD2 [order 2] : [VENT_CMP_DETECT==true]
  VVIR_REF_PERIOD2 -> Refractory_VVIR1 [order 1] : [VENT_CMP_DETECT==true]
  Refractory_VVIR1 -> VVIR_REF_PERIOD2 : after(VENT_Refractory_Period,msec)
  VVIR_REF_PERIOD2 -> VVIR [order 2] : after(60000/Adaptive_Rate-VENT_Refractory_Period,msec)
  VVI_REF_PERIOD2 -> VVI_LED1 : after(VENT_Refractory_Period,msec)
  pacing_VVIR -> Refractory_VVIR : after(VENT_Pulse_Width,msec)
  VVIR_REF_PERIOD1 -> VVIR [order 1] : after(60000/Adaptive_Rate-VENT_Refractory_Period-VENT_Pulse_Width,msec)
  VVI_LED -> VVI_REF_PERIOD2 [order 1] : [VENT_CMP_DETECT==true]
  VVI_REF_PERIOD1 -> VVI_LED : after(VENT_Refractory_Period,msec)
  VVIR_REF_PERIOD1 -> Refractory_VVIR1 [order 2] : [VENT_CMP_DETECT==true]
  Refractory_VVIR -> VVIR_REF_PERIOD1 : after(VENT_Refractory_Period,msec)
  DOO -> pacing_DOO_ATR [order 1] : after(60000/Lower_Rate_Limit -VENT_Pulse_Width-AV_Delay,msec)
  pacing_DOO_ATR -> DOO_Vcharge_Adischarge : after(ATR_Pulse_Width,msec)
  DOOR -> pacing_DOOR_ATR [order 1] : after(60000/Adaptive_Rate -VENT_Pulse_Width-AV_Delay,msec)
  DOO_VENT -> DOO : after(VENT_Pulse_Width,msec)
  pacing_DOOR_ATR -> DOOR_Vcharge_Adischarge : after(ATR_Pulse_Width,msec)
  DOOR_VENT -> DOOR : after(VENT_Pulse_Width,msec)
  DOO_Vcharge_Adischarge -> DOO_VENT : after(AV_Delay-ATR_Pulse_Width,msec)
  DOOR_Vcharge_Adischarge -> DOOR_VENT : after(AV_Delay-ATR_Pulse_Width,msec)
  data: PACE_GND_CTRL output boolean; ATR_PACE_CTRL output boolean; Current_Pace_Amp output uint16; PACE_CHARGE_CTRL output boolean; ATR_GND_CTRL output boolean; VENT_PACE_CTRL output boolean; VENT_GND_CTRL output boolean; FRONTEND_CTRL output boolean; Z_ATR_CTRL output boolean; Z_VENT_CTRL output boolean; ATR_CMP_DETECT input boolean; VENT_CMP_DETECT input boolean; Lower_Rate_Limit input uint16; ATR_Pulse_Width input uint16; VENT_Pulse_Width input uint16; ATR_Refractory_Period input uint16; VENT_Refractory_Period input uint16; ATR_Amp input uint16; AV_Delay input uint16; VENT_Amp input uint16; setmode input; Adaptive_Rate input uint16; LED_GREEN output

== stateflow chart Part1_Simulink/Serial_Inputs ==
  settings: executeAtInitialization=1
  state SET_PARAM
    entry:
    %red_enable= false;
    %blue_enable= true;
    setmode= typecast(rxdata(3:4),'uint16');
    Lower_Rate_Limit = typecast(rxdata(5:6),'uint16');
    ATR_Pulse_Width = typecast(rxdata(7:8),'uint16');
    VENT_Pulse_Width= typecast(rxdata(9:10),'uint16');
    ATR_Refractory_Period=typecast(rxdata(11:12),'uint16');
    VENT_Refractory_Period=typecast(rxdata(13:14),'uint16');
    ATR_Amp =typecast(rxdata(15:16),'uint16');
    VENT_Amp=typecast(rxdata(17:18),'uint16');
    Response_factor=typecast(rxdata(19:20),'uint16');
    MaxSensorate=typecast(rxdata(21:22),'uint16');
    AV_delay=typecast(rxdata(23:24),'uint16');
    Activity_threshold=typecast(rxdata(25:26),'uint16');
    VENT_Sensitivity=typecast(rxdata(27:34),'double');
    ATR_Sensitivity=typecast(rxdata(35:42),'double');
  state Send_Param1
    entry:
    %red_enable= true;
    %LED_RED=true;
    if VENT_Amp == uint16(0)
    LED_RED = true;
    end
    LED_BLUE= false;
    send_params();
  state INITIAL
    %set the initial values of parameter
    entry:
    %red_enable = true;
    %blue_enable = false;
    %uint16
    LED_BLUE=false;
    setmode=4;
    Lower_Rate_Limit = 60;
    ATR_Pulse_Width = 5;
    VENT_Pulse_Width=5;
    ATR_Refractory_Period = 250;
    VENT_Refractory_Period= 320;
    ATR_Amp = 75;
    VENT_Amp= 75;
    Response_factor=30;
    MaxSensorate=120;
    AV_delay=150;
    Activity_threshold = 1;
    ID = 11;
  state STANDBY
    %standby
  state Send_Param
    entry:
    %red_enable= true;
    LED_RED=false;
    LED_BLUE= true;
    send_params();
  SET_PARAM -> Send_Param1
  (default) -> INITIAL
  (junction 82) -> SET_PARAM [order 1] : [rxdata(2) == hex2dec('55')]
  (junction 80) -> STANDBY [order 2]
  Send_Param1 -> STANDBY
  INITIAL -> STANDBY
  STANDBY -> (junction 80) : [status==0]
  (junction 80) -> (junction 82) [order 1] : [rxdata(1) == hex2dec('16')]
  (junction 82) -> Send_Param [order 2] : [rxdata(2) == hex2dec('22')]
  Send_Param -> STANDBY
  data: Lower_Rate_Limit output uint16; ATR_Pulse_Width output uint16; VENT_Pulse_Width output uint16; ATR_Refractory_Period output uint16; VENT_Refractory_Period output uint16; ATR_Amp output uint16; VENT_Amp output uint16; rxdata input uint8; AV_delay output uint16; Activity_threshold output uint16; Response_factor output uint16; MaxSensorate output uint16; setmode output uint16; VENT_Sensitivity output double; ATR_Sensitivity output double; ID output uint16; LED_BLUE output; LED_RED output; status input uint8
